simulink model "test"  (Simulink 7.4)
settings: Solver=ode45  StartTime=0.0  StopTime=10  RelTol=1e-3
values from neighbouring files (symbols this model uses):
  Bs = 1.748817703686052e-04    (= 0.000174881770369)    [armposregdimensionering.m]    (also in armposregsimuStart.m; hastighedsreguleringStart.m; hastregDimensionering.m; pindposregdimensionering.m)
  g = 9.816    [armposregsimuStart.m]    (also in hastighedsreguleringStart.m; pindposregdimensionering.m = 9.82; pindregStart.m)
  initU = 1.7    [armposregsimuStart.m]    (also in hastighedsreguleringStart.m; pindregStart.m)
  Js = 2.686970843428432e-04    (= 0.000268697084343)    [armposregdimensionering.m]    (also in armposregsimuStart.m; hastighedsreguleringStart.m; hastregDimensionering.m; pindposregdimensionering.m)
  kff = (3*la)/(2*lp)    [pindregStart.m]
  kipp = 1    [pindposregdimensionering.m]
  Km = 0.022141706562986    (= 0.022141706563)    [armposregdimensionering.m]    (also in armposregsimuStart.m; hastighedsreguleringStart.m; hastregDimensionering.m; pindposregdimensionering.m)
  Kpg = 236    [armposregdimensionering.m]
  Kpim = 0.2    [armposregdimensionering.m]    (also in hastregDimensionering.m)
  la = 0.3384    [armposregdimensionering.m]    (also in armposregsimuStart.m; hastighedsreguleringStart.m; hastregDimensionering.m; pindposregdimensionering.m)
  lp = 1.1509    [armposregsimuStart.m]    (also in hastighedsreguleringStart.m; pindposregdimensionering.m; pindregStart.m)
  ma = 0.2988    [armposregdimensionering.m]    (also in armposregsimuStart.m = 0.298; hastighedsreguleringStart.m = 0.298; hastregDimensionering.m; pindposregdimensionering.m)
  N = 12/40    (= 0.3)    [armposregdimensionering.m]    (also in armposregsimuStart.m; hastighedsreguleringStart.m; hastregDimensionering.m; pindposregdimensionering.m)
  Rm = 0.807790757873553    (= 0.807790757874)    [armposregdimensionering.m]    (also in armposregsimuStart.m; hastighedsreguleringStart.m; hastregDimensionering.m; pindposregdimensionering.m)
  tauf = 0.064    [armposregsimuStart.m]    (also in pindregStart.m)
undefined symbols (not defined in the file or in its folder): kd, ki
libraries: vrlib x3
settings Model: Creator=Skov  LastModifiedBy=HOSTRUP

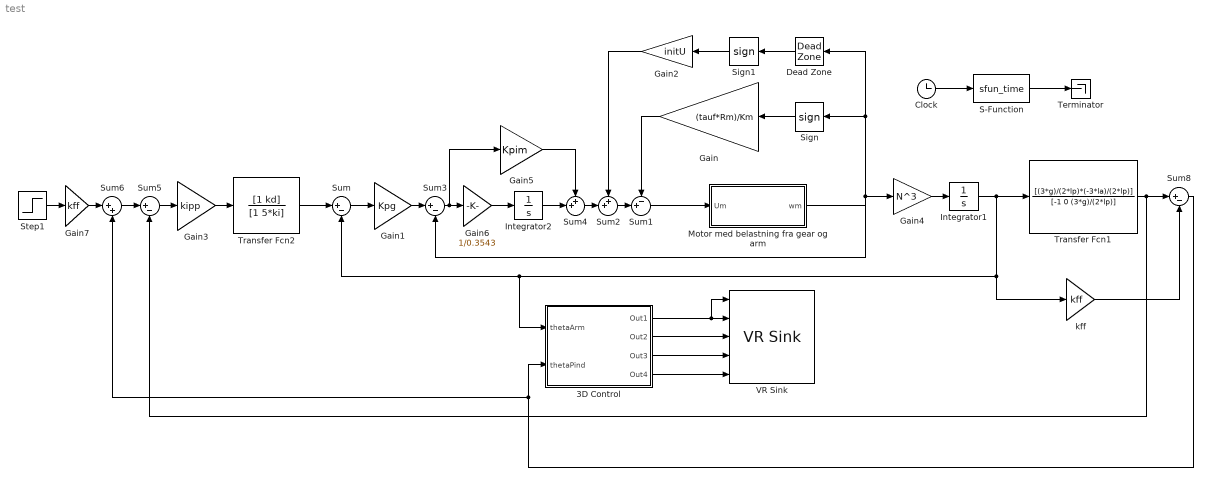
== system test ==
  3D Control : Subsystem
  Clock : Clock
      settings: Decimation=10
  Dead Zone : DeadZone  LowerValue=-0.1  UpperValue=0.1  SaturateOnIntegerOverflow=on
  Gain : Gain  Gain=(tauf*Rm)/Km  ParameterDataType=fixdt(1, 16)  ParameterScaling=2^0  OutDataType=fixdt(1, 16)  OutScaling=2^0
  Gain1 : Gain  Gain=Kpg  ParameterDataType=fixdt(1, 16)  ParameterScaling=2^0  OutDataType=fixdt(1, 16)  OutScaling=2^0
  Gain2 : Gain  Gain=initU  ParameterDataType=fixdt(1, 16)  ParameterScaling=2^0  OutDataType=fixdt(1, 16)  OutScaling=2^0
  Gain3 : Gain  Gain=kipp  ParameterDataType=fixdt(1, 16)  ParameterScaling=2^0  OutDataType=fixdt(1, 16)  OutScaling=2^0
  Gain4 : Gain  Gain=N^3  ParameterDataType=fixdt(1, 16)  ParameterScaling=2^0  OutDataType=fixdt(1, 16)  OutScaling=2^0
  Gain5 : Gain  Gain=Kpim  ParameterDataType=fixdt(1, 16)  ParameterScaling=2^0  OutDataType=fixdt(1, 16)  OutScaling=2^0
  Gain6 : Gain  Gain=1/0.3543  ParameterDataType=fixdt(1, 16)  ParameterScaling=2^0  OutDataType=fixdt(1, 16)  OutScaling=2^0
  Gain7 : Gain  Gain=kff  ParameterDataType=fixdt(1, 16)  ParameterScaling=2^0  OutDataType=fixdt(1, 16)  OutScaling=2^0
  Integrator1 : Integrator
  Integrator2 : Integrator
  Motor med belastning fra gear og arm : Subsystem
  S-Function : S-Function  FunctionName=sfun_time  EnableBusSupport=off
  Sign : Signum  SampleTime=0.01
  Sign1 : Signum
  Step1 : Step  After=pi/18  SampleTime=0
  Sum{,3,5,8} (4 alike) : Sum  Inputs=|+-  OutDataType=fixdt(1, 16)  OutScaling=2^0
  Sum1 : Sum  Inputs=-+|  OutDataType=fixdt(1, 16)  OutScaling=2^0
  Sum2 : Sum  Inputs=++|  OutDataType=fixdt(1, 16)  OutScaling=2^0
  Sum4 : Sum  Inputs=++|  OutDataType=fixdt(1, 16)  OutScaling=2^0
  Sum6 : Sum  Inputs=|++  OutDataType=fixdt(1, 16)  OutScaling=2^0
  Terminator : Terminator
  Transfer Fcn1 : TransferFcn  Numerator=[(3*g)/(2*lp)*(-3*la)/(2*lp)]  Denominator=[-1 0 (3*g)/(2*lp)]
  Transfer Fcn2 : TransferFcn  Numerator=[1 kd]  Denominator=[1 5*ki]
  VR Sink : vrlib/VR Sink  InstantiateOnLoad=on  SampleTime=0.02  ViewEnable=on  RemoteChange=off  RemoteView=on  FieldsWritten=Ball.rotation.4.1.double#Arm.rotation.4.1.double#Pind.translation.3.1.double#AP.translation.3.1.double#Pind.rotation.4.1.double  WorldFileName=VRML1.WRL  AutoView=off  VideoDimensions=[]  FigureProperties="{'Position', 'Name', 'Viewpoint', 'CameraBound', 'CameraDirection', 'CameraPosition', 'CameraUpVector', 'ZoomFactor', 'Antialiasing', 'Headlight', 'Lighting', 'NavPanel', 'StatusBar', 'ToolBar', 'Textures', 'Transparency', 'Wireframe', 'NavZones', 'NavMode', 'NavSpeed', 'Record2DCompressMethod', 'Record2DCompressQuality', 'Record2D', 'Record2DFileName', 'Record2DFPS'; [3.8900000000000000e+002  1.2070000000000000e+003  5.7600000000000000e+002  3.8000000000000000e+002], '', '', 'on', [0.0000000000000000e+000  0.0000000000000000e+000 -1.0000000000000000e+000], [0.0000000000000000e+000  0.0000000000000000e+000  1.0000000000000000e+001], [0.0000000000000000e+000  1.0000000000000000e+000  0.0000000000000000e+000], [1.0000000000000000e+000], 'off', 'on', 'on', 'halfbar', 'on', 'on', 'on', 'on', 'off', 'off', 'fly', 'normal', 'auto', [7.5000000000000000e+001], 'off', '%f_anim_%n.avi', [1.5000000000000000e+001]}"
  kff : Gain  Gain=kff  ParameterDataType=fixdt(1, 16)  ParameterScaling=2^0  OutDataType=fixdt(1, 16)  OutScaling=2^0
  wires:
  Sign/1 -> Gain/1
  Gain4/1 -> Integrator1/1
  Integrator1/1 -> Transfer Fcn1/1, 3D Control/1(thetaArm), Sum/2, kff/1
  Gain1/1 -> Sum3/1
  Sum/1 -> Gain1/1
  S-Function/1 -> Terminator/1
  Clock/1 -> S-Function/1
  Sum2/1 -> Sum1/2
  Dead Zone/1 -> Sign1/1
  Sign1/1 -> Gain2/1
  Transfer Fcn2/1 -> Sum/1
  Motor med belastning fra gear og arm/1(wm) -> Sign/1, Dead Zone/1, Sum3/2, Gain4/1
  3D Control/1(Out1) -> VR Sink/1, VR Sink/2
  3D Control/2(Out2) -> VR Sink/3
  3D Control/3(Out3) -> VR Sink/4
  3D Control/4(Out4) -> VR Sink/5
  Gain6/1 -> Integrator2/1
  Integrator2/1 -> Sum4/2
  Gain5/1 -> Sum4/1
  Sum4/1 -> Sum2/2
  Sum3/1 -> Gain6/1, Gain5/1
  Sum1/1 -> Motor med belastning fra gear og arm/1(Um)
  Gain/1 -> Sum1/1
  Gain2/1 -> Sum2/1
  Transfer Fcn1/1 -> Sum8/1, Sum5/2
  kff/1 -> Sum8/2
  Sum8/1 -> 3D Control/2(thetaPind), Sum6/2
  Sum6/1 -> Sum5/1
  Gain7/1 -> Sum6/1
  Step1/1 -> Gain7/1
  Sum5/1 -> Gain3/1
  Gain3/1 -> Transfer Fcn2/1

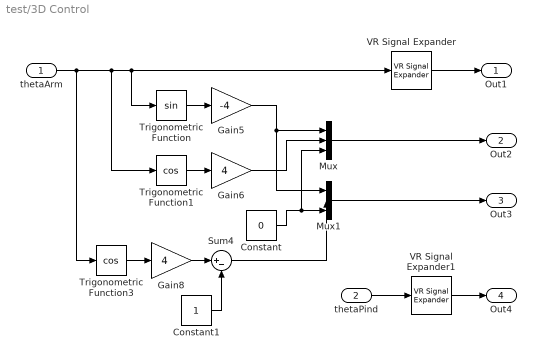
== system test/3D Control ==
  thetaArm : Inport  OutDataType=fixdt(1, 16)  OutScaling=2^0
  thetaPind : Inport  Port=2  OutDataType=fixdt(1, 16)  OutScaling=2^0
  Constant : Constant  Value=0  OutDataType=fixdt(1, 16)  OutScaling=2^0
  Constant1 : Constant  OutDataType=fixdt(1, 16)  OutScaling=2^0
  Gain5 : Gain  Gain=-4  ParameterDataType=fixdt(1, 16)  ParameterScaling=2^0  OutDataType=fixdt(1, 16)  OutScaling=2^0
  Gain6 : Gain  Gain=4  ParameterDataType=fixdt(1, 16)  ParameterScaling=2^0  OutDataType=fixdt(1, 16)  OutScaling=2^0
  Gain8 : Gain  Gain=4  ParameterDataType=fixdt(1, 16)  ParameterScaling=2^0  OutDataType=fixdt(1, 16)  OutScaling=2^0
  Mux : Mux  Inputs=3
  Mux1 : Mux  Inputs=3
  Sum4 : Sum  Inputs=|+-  OutDataType=fixdt(1, 16)  OutScaling=2^0
  Trigonometric Function : Trigonometry
  Trigonometric Function1 : Trigonometry  Operator=cos
  Trigonometric Function3 : Trigonometry  Operator=cos
  VR Signal Expander : vrlib/VR Signal Expander  SystemSampleTime=-1  outwidth=4  outidx=[4]
  VR Signal Expander1 : vrlib/VR Signal Expander  SystemSampleTime=-1  outwidth=4  outidx=[4]
  Out1 : Outport  OutDataType=fixdt(1, 16)  OutScaling=2^0
  Out2 : Outport  Port=2  OutDataType=fixdt(1, 16)  OutScaling=2^0
  Out3 : Outport  Port=3  OutDataType=fixdt(1, 16)  OutScaling=2^0
  Out4 : Outport  Port=4  OutDataType=fixdt(1, 16)  OutScaling=2^0
  wires:
  VR Signal Expander/1 -> Out1/1
  Trigonometric Function/1 -> Gain5/1
  Gain5/1 -> Mux/1, Mux1/1
  Trigonometric Function1/1 -> Gain6/1
  Gain6/1 -> Mux/2
  Constant/1 -> Mux/3, Mux1/3
  Mux/1 -> Out2/1
  Trigonometric Function3/1 -> Gain8/1
  Gain8/1 -> Sum4/1
  Constant1/1 -> Sum4/2
  Sum4/1 -> Mux1/2
  Mux1/1 -> Out3/1
  VR Signal Expander1/1 -> Out4/1
  thetaPind/1 -> VR Signal Expander1/1
  thetaArm/1 -> VR Signal Expander/1, Trigonometric Function/1, Trigonometric Function1/1, Trigonometric Function3/1

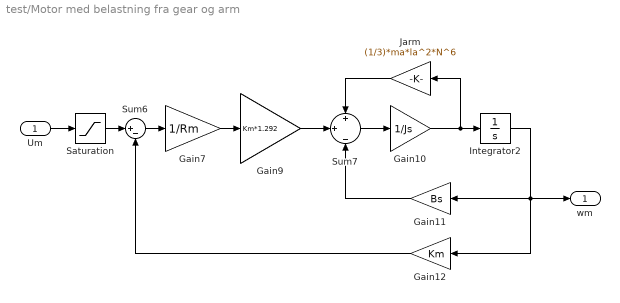
== system test/Motor med belastning fra gear og arm ==
  Um : Inport  OutDataType=fixdt(1, 16)  OutScaling=2^0
  Gain10 : Gain  Gain=1/Js  ParameterDataType=fixdt(1, 16)  ParameterScaling=2^0  OutDataType=fixdt(1, 16)  OutScaling=2^0
  Gain11 : Gain  Gain=Bs  ParameterDataType=fixdt(1, 16)  ParameterScaling=2^0  OutDataType=fixdt(1, 16)  OutScaling=2^0
  Gain12 : Gain  Gain=Km  ParameterDataType=fixdt(1, 16)  ParameterScaling=2^0  OutDataType=fixdt(1, 16)  OutScaling=2^0
  Gain7 : Gain  Gain=1/Rm  ParameterDataType=fixdt(1, 16)  ParameterScaling=2^0  OutDataType=fixdt(1, 16)  OutScaling=2^0
  Gain9 : Gain  Gain=Km*1.292  ParameterDataType=fixdt(1, 16)  ParameterScaling=2^0  OutDataType=fixdt(1, 16)  OutScaling=2^0
  Integrator2 : Integrator
  Jarm : Gain  Gain=(1/3)*ma*la^2*N^6  ParameterDataType=fixdt(1, 16)  ParameterScaling=2^0  OutDataType=fixdt(1, 16)  OutScaling=2^0
  Saturation : Saturate  UpperLimit=10  LowerLimit=-10  OutDataType=fixdt(1, 16)  OutScaling=2^0
  Sum6 : Sum  Inputs=|+-  OutDataType=fixdt(1, 16)  OutScaling=2^0
  Sum7 : Sum  Inputs=+|+|-  OutDataType=fixdt(1, 16)  OutScaling=2^0
  wm : Outport  OutDataType=fixdt(1, 16)  OutScaling=2^0
  wires:
  Sum6/1 -> Gain7/1
  Gain7/1 -> Gain9/1
  Gain10/1 -> Integrator2/1, Jarm/1
  Sum7/1 -> Gain10/1
  Integrator2/1 -> Gain11/1, Gain12/1, wm/1
  Gain12/1 -> Sum6/2
  Saturation/1 -> Sum6/1
  Um/1 -> Saturation/1
  Gain11/1 -> Sum7/3
  Jarm/1 -> Sum7/1
  Gain9/1 -> Sum7/2
